simulink model "DiscreteAtomicTest"  (R2017a)
settings: Solver=FixedStepAuto  StartTime=0.0  StopTime=.2  FixedStep=1e-7  RelTol=1e-3
undefined symbols (not defined in the file or in its folder): DiscIntNeverNeededParam
settings Model: Creator=erich  LastModifiedBy=erich

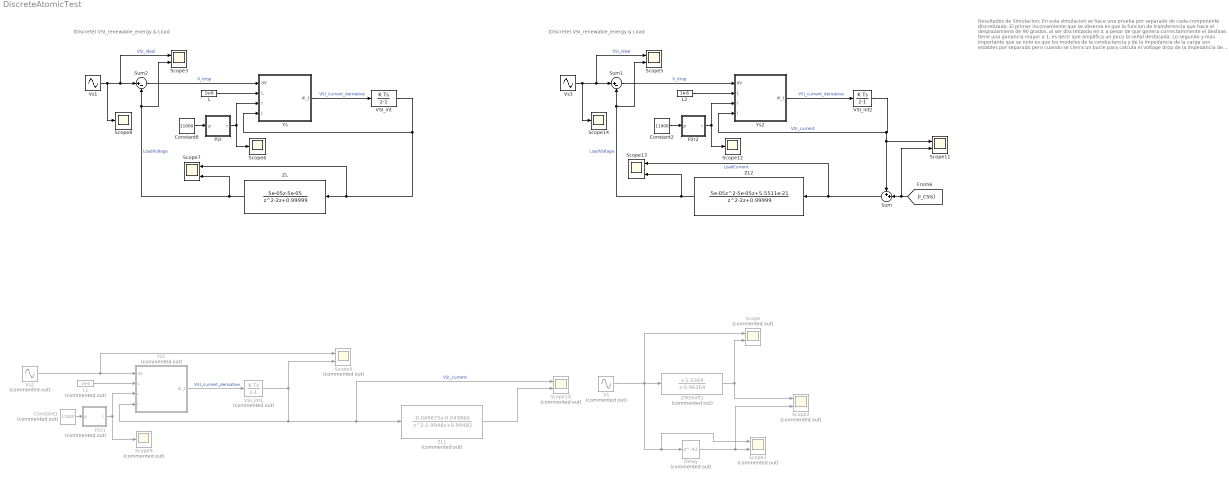
== system DiscreteAtomicTest ==
  note: Resultados de Simulacion:
      | En esta simulacion se hace una prueba por separado de cada componente discretizado.
      | El primer inconveniente que se observa es que la funcion de transferencia que hace
      | el desplazamieno de 90 grados, al ser discretizada en z, a pesar de que genera correctammente
      | el desfase, tiene una ganancia mayor a 1, es decir que amplifica un poco la señal desfasada.
      |
      | Lo segundo y mas importante que se noto es que los modelos de la conductancia y de la
      | impedancia de la carga son estables por separado pero cuando se cierra un bucle para
      | calcula el voltage drop de la impedancia de linea de Vs, el sistema se vuelve inestable
      |
      | como resultado de todo esto tome la decicion de expresar el modelo de una manera diferente.
      | tanto la carga como la conductancia seran expresadas usando una unica matlabfunction
      | la cual implementara un sistema de ecuaciones diferenciales acopladas.
      |
      | finalmente cabe agregar que la inestabilidad se observo para pasos de simmulacion de
      | 1e-3 1e-4 y 1e-7 y usando 2 metodos diferentes, zoh y invariante al impulso.
  note: (Discrete) VSI_renewable_energy & Load
  note: (Discrete) VSI_renewable_energy & Load
  Constant1 : Constant  Commented=on  Value=11000
  Constant2 : Constant  Value=11000
  Constant8 : Constant  Value=11000
  Delay : Delay  Commented=on  DelayLength=42
  L : Constant  Value=1e-6
  L1 : Constant  Commented=on  Value=1e-6
  L2 : Constant  Value=1e-6
  P2r : MATLAB Function  TreatAsAtomicUnit=on  SystemSampleTime=1e-07
  P2r1 : MATLAB Function  Commented=on  TreatAsAtomicUnit=on  SystemSampleTime=0.0001
  P2r2 : MATLAB Function  TreatAsAtomicUnit=on  SystemSampleTime=1e-07
  Scope{,1..2,4,10} (5 alike) : Scope  Commented=on  NumInputPorts=2
  Scope{3,5,7,11,13} (5 alike) : Scope  NumInputPorts=2
  Scope{6,8,12,14} (4 alike) : Scope
  Scope9 : Scope  Commented=on
  Sum : Sum  Inputs=++|
  Sum1 : Sum  Inputs=|+-
  Sum2 : Sum  Inputs=|+-
  VSI_int : DiscreteIntegrator  InitialConditionSetting=State (most efficient)  SampleTime=1e-07  UpperSaturationLimit=1000  LowerSaturationLimit=-1000  ICPrevOutput=DiscIntNeverNeededParam  ICPrevScaledInput=DiscIntNeverNeededParam
  VSI_int1 : DiscreteIntegrator  Commented=on  InitialConditionSetting=State (most efficient)  SampleTime=0.0001  ICPrevOutput=DiscIntNeverNeededParam  ICPrevScaledInput=DiscIntNeverNeededParam
  VSI_int2 : DiscreteIntegrator  InitialConditionSetting=State (most efficient)  SampleTime=1e-07  ICPrevOutput=DiscIntNeverNeededParam  ICPrevScaledInput=DiscIntNeverNeededParam
  Vs : Sin  Commented=on  Amplitude=170  Frequency=2*pi*60  SampleTime=1e-04
  Vs1 : Sin  Amplitude=170  Frequency=2*pi*60  SampleTime=1e-07
  Vs2 : Sin  Commented=on  Amplitude=.1  Frequency=2*pi*60  SampleTime=0.0001
  Vs3 : Sin  Amplitude=170  Frequency=2*pi*60  SampleTime=1e-07
  Ys : MATLAB Function  TreatAsAtomicUnit=on  SystemSampleTime=1e-07
      settings: MinAlgLoopOccurrences=on
  Ys1 : MATLAB Function  Commented=on  TreatAsAtomicUnit=on  SystemSampleTime=0.0001
      settings: MinAlgLoopOccurrences=on
  Ys2 : MATLAB Function  TreatAsAtomicUnit=on  SystemSampleTime=1e-07
      settings: MinAlgLoopOccurrences=on
  Z90Shift1 : DiscreteTransferFcn  Commented=on  Numerator="[1     -1.0364]"  Denominator="[1    -0.96364]"
  ZL : DiscreteTransferFcn  Numerator="[0       5e-05      -5e-05]"  Denominator="[1          -2     0.99999]"  SampleTime=1e-7  a0EqualsOne=on
  ZL1 : DiscreteTransferFcn  Commented=on  Numerator="[0    0.049875   -0.049866]"  Denominator="[1     -1.9948     0.99482]"
  ZL2 : DiscreteTransferFcn  Numerator="[5e-05      -5e-05  5.5511e-21]"  Denominator="[1          -2     0.99999]"
  wires:
  Vs/1 -> Scope1/1, Delay/1, Z90Shift1/1, Scope/1
  Z90Shift1/1 -> Scope/2, Scope2/1
  Delay/1 -> Scope2/2, Scope1/2
  L1/1 -> Ys1/2(L)
  P2r1/1(r) -> Ys1/3(r), Scope9/1
  VSI_int1/1 -> Ys1/4(I), Scope10/1, ZL1/1, Scope4/2  "VSI_current"
  Ys1/1(dI_t) -> VSI_int1/1  "VSI_current_derivative"
  Constant1/1 -> P2r1/1(p)
  Vs2/1 -> Scope4/1, Ys1/1(dV)
  ZL1/1 -> Scope10/2
  Sum2/1 -> Ys/1(dV)  "V_drop"
  VSI_int/1 -> Ys/4(I), Scope7/1, ZL/1
  L/1 -> Ys/2(L)
  Constant8/1 -> P2r/1(p)
  ZL/1 -> Scope7/2, Scope3/2, Sum2/2  "LoadVoltage"
  Vs1/1 -> Scope8/1, Scope3/1, Sum2/1  "VSI_ideal"
  Ys/1(dI_t) -> VSI_int/1  "VSI_current_derivative"
  P2r/1(r) -> Ys/3(r), Scope6/1
  Sum1/1 -> Ys2/1(dV)  "V_drop"
  Sum/1 -> Scope13/1, ZL2/1  "LoadCurrent"
  L2/1 -> Ys2/2(L)
  Constant2/1 -> P2r2/1(p)
  ZL2/1 -> Scope13/2, Scope5/2, Sum1/2  "LoadVoltage"
  Vs3/1 -> Scope14/1, Scope5/1, Sum1/1  "VSI_ideal"
  VSI_int2/1 -> Ys2/4(I), Scope11/1, Sum/1  "VSI_current"
  [I_CSIs] -> Scope11/2, Sum/2
  Ys2/1(dI_t) -> VSI_int2/1  "VSI_current_derivative"
  P2r2/1(r) -> Ys2/3(r), Scope12/1

== matlab function DiscreteAtomicTest/P2r1 ==
  data: p input; r output
function r = fcn(p)

x = 1e-3;

if(p>7000)
    x=1e-3;
end

if(p<=7000 && p>1000)
    x=100e-3;
end

if(p<=1000)
    x=.5;
end

r = x;

== matlab function DiscreteAtomicTest/P2r2 ==
  data: p input; r output
function r = fcn(p)

x = 1e-3;

if(p>7000)
    x=1e-3;
end

if(p<=7000 && p>1000)
    x=100e-3;
end

if(p<=1000)
    x=.5;
end

r = x;

== matlab function DiscreteAtomicTest/Ys1 ==
  data: dV input; dI_t output; L input; r input; I input
function dI_t = fcn(dV, L, r, I)

dI_t = dV/L - I*r/(L);

== matlab function DiscreteAtomicTest/Ys2 ==
  data: dV input; dI_t output; L input; r input; I input
function dI_t = fcn(dV, L, r, I)

dI_t = dV/L - I*r/(L);

== matlab function DiscreteAtomicTest/Ys ==
  data: dV input; dI_t output; L input; r input; I input
function dI_t = fcn(dV, L, r, I)

dI_t = dV/L - I*r/(L);

== matlab function DiscreteAtomicTest/P2r ==
  data: p input; r output
function r = fcn(p)

x = 1e-3;

if(p>7000)
    x=1e-3;
end

if(p<=7000 && p>1000)
    x=100e-3;
end

if(p<=1000)
    x=.5;
end

r = x;
